simulink model "s3"  (R2025b)
settings: Solver=VariableStepAuto  StartTime=0.0  StopTime=10  RelTol=1e-3
undefined symbols (not defined in the file): X, Y, Z
libraries: nesl_utility x21, sm_lib x20, robotcorelib x1, simulink x1
settings Model: Creator=lucaa  LastModifiedBy=antoniozerbato

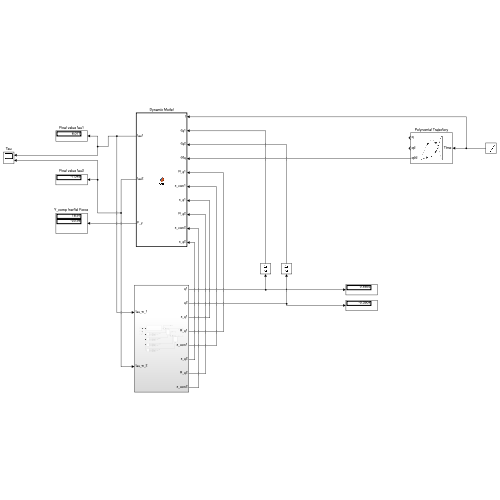
[thumbnail: Simulink's stored preview of the top-level diagram]
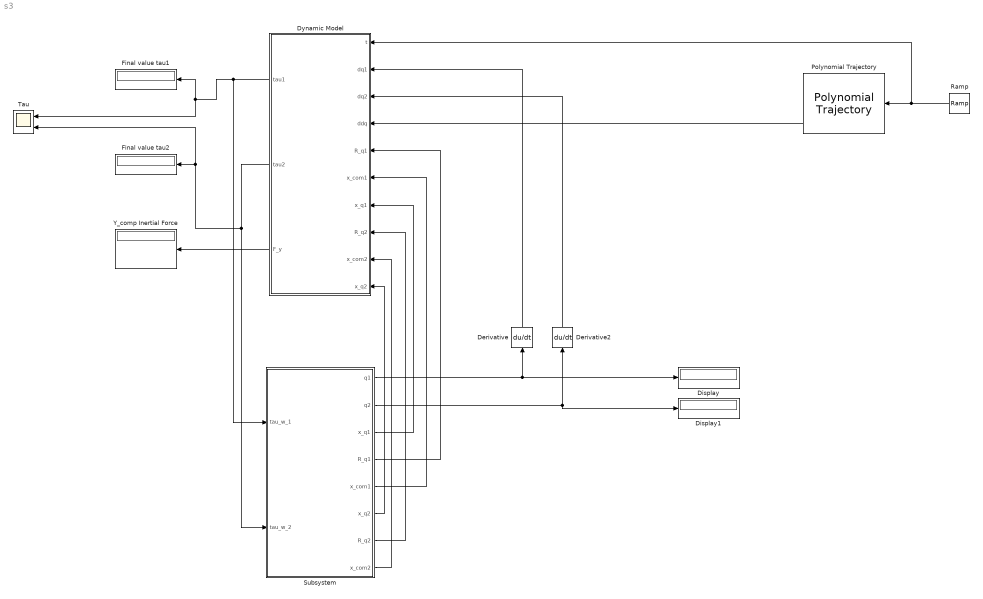
== system s3 ==
  Derivative : Derivative
  Derivative2 : Derivative
  Display : Display
  Display1 : Display
  Dynamic Model : MATLAB Function  TreatAsAtomicUnit=on
  Final value tau1 : Display
  Final value tau2 : Display
  Polynomial Trajectory : robotcorelib/Polynomial Trajectory  WaypointSource=Internal  Waypoints=[pi/36,pi*(4/18);-pi*(3/36),-pi/9]  TimePoints=[0,10]  TimeInterval=[ 1, 4 ]  Method=Cubic Polynomial  ParameterSource=Internal  VelocityBoundaryCondition=zeros( 2,2 )  AccelerationBoundaryCondition=zeros( 2, 5 )  SimulateUsing=Interpreted execution
  Ramp : simulink/Sources/Ramp  slope=1  start=0  InitialOutput=0
  Subsystem : Subsystem
  Tau : Scope  NumInputPorts=2
      settings: ActiveDisplayYMinimum=-0.050415777209954854  ActiveDisplayYMaximum=0.012289469598716157
  "Y_comp Inertial Force " : Display
  wires:
  Dynamic Model/1(tau1) -> Subsystem/1(tau_w_1), Final value tau1/1, Tau/1
  Dynamic Model/2(tau2) -> Subsystem/2(tau_w_2), Final value tau2/1, Tau/2
  Polynomial Trajectory/3 -> Dynamic Model/4(ddq)
  Ramp/1 -> Polynomial Trajectory/1, Dynamic Model/1(t)
  Dynamic Model/3(F_y) -> "Y_comp Inertial Force "/1
  Derivative/1 -> Dynamic Model/2(dq1)
  Derivative2/1 -> Dynamic Model/3(dq2)
  Subsystem/6(x_q2) -> Dynamic Model/10(x_q2)
  Subsystem/8(x_com2) -> Dynamic Model/9(x_com2)
  Subsystem/7(R_q2) -> Dynamic Model/8(R_q2)
  Subsystem/3(x_q1) -> Dynamic Model/7(x_q1)
  Subsystem/1(q1) -> Derivative/1, Display/1
  Subsystem/2(q2) -> Derivative2/1, Display1/1
  Subsystem/5(x_com1) -> Dynamic Model/6(x_com1)
  Subsystem/4(R_q1) -> Dynamic Model/5(R_q1)

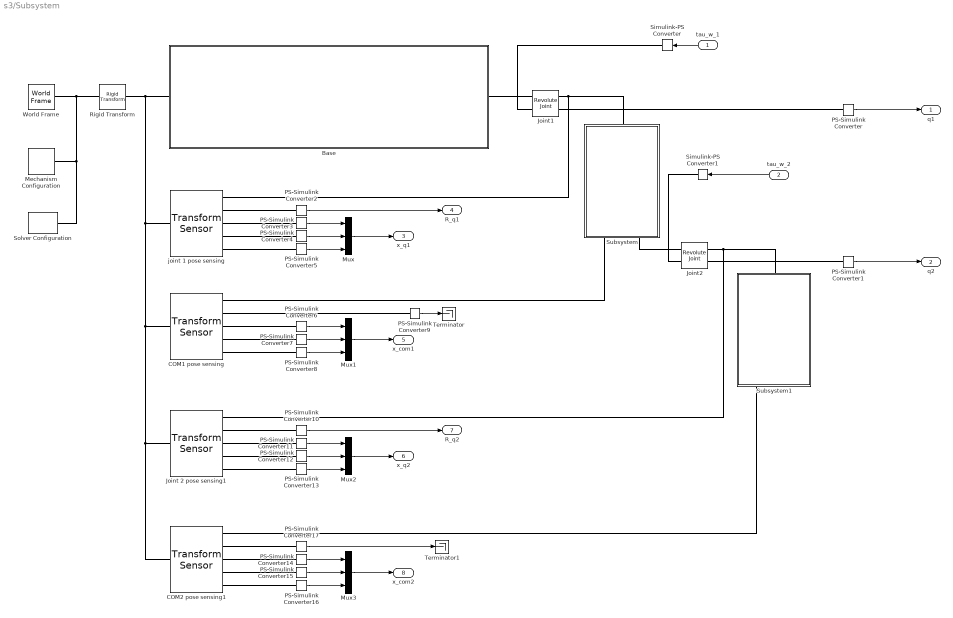
== system s3/Subsystem ==
  tau_w_1 : Inport
  tau_w_2 : Inport  Port=2
  " Joint1" : sm_lib/Joints/Revolute Joint  JointMode=Normal  CompositeWrenchDir=FollowerOnBase  CompositeWrenchFrame=BaseFrame  SenseConstraintForce=off  SenseConstraintTorque=off  SenseTotalForce=off  SenseTotalTorque=off  PositionTargetSpecify=on  PositionTargetPriority=High  PositionTargetValue=5  PositionTargetValueUnits=deg  VelocityTargetSpecify=off  VelocityTargetPriority=High  VelocityTargetValue=0  VelocityTargetValueUnits=deg/s  EquilibriumPosition=0  EquilibriumPositionUnits=deg  SpringStiffness=0  SpringStiffnessUnits=N*m/deg  DampingCoefficient=0  DampingCoefficientUnits=N*m/(deg/s)  LowerLimitSpecify=off  LowerLimitBound=-90  LowerLimitBoundUnits=deg  LowerLimitStiffness=1e4  LowerLimitStiffnessUnits=N*m/deg  LowerLimitDamping=10  LowerLimitDampingUnits=N*m/(deg/s)  LowerLimitTransitionRegionWidth=0.1  LowerLimitTransitionRegionWidthUnits=deg  UpperLimitSpecify=off  UpperLimitBound=90  UpperLimitBoundUnits=deg  UpperLimitStiffness=1e4  UpperLimitStiffnessUnits=N*m/deg  UpperLimitDamping=10  UpperLimitDampingUnits=N*m/(deg/s)  UpperLimitTransitionRegionWidth=0.1  UpperLimitTransitionRegionWidthUnits=deg  TorqueActuationMode=InputTorque  MotionActuationMode=ComputedMotion  SensePosition=on  SenseVelocity=off  SenseAcceleration=off  SenseTorqueForce=off  SenseLowerLimitTorqueForce=off  SenseUpperLimitTorqueForce=off
  " Joint2" : sm_lib/Joints/Revolute Joint  JointMode=Normal  CompositeWrenchDir=FollowerOnBase  CompositeWrenchFrame=BaseFrame  SenseConstraintForce=off  SenseConstraintTorque=off  SenseTotalForce=off  SenseTotalTorque=off  PositionTargetSpecify=on  PositionTargetPriority=High  PositionTargetValue=-15  PositionTargetValueUnits=deg  VelocityTargetSpecify=off  VelocityTargetPriority=High  VelocityTargetValue=0  VelocityTargetValueUnits=deg/s  EquilibriumPosition=0  EquilibriumPositionUnits=deg  SpringStiffness=0  SpringStiffnessUnits=N*m/deg  DampingCoefficient=0  DampingCoefficientUnits=N*m/(deg/s)  LowerLimitSpecify=off  LowerLimitBound=-90  LowerLimitBoundUnits=deg  LowerLimitStiffness=1e4  LowerLimitStiffnessUnits=N*m/deg  LowerLimitDamping=10  LowerLimitDampingUnits=N*m/(deg/s)  LowerLimitTransitionRegionWidth=0.1  LowerLimitTransitionRegionWidthUnits=deg  UpperLimitSpecify=off  UpperLimitBound=90  UpperLimitBoundUnits=deg  UpperLimitStiffness=1e4  UpperLimitStiffnessUnits=N*m/deg  UpperLimitDamping=10  UpperLimitDampingUnits=N*m/(deg/s)  UpperLimitTransitionRegionWidth=0.1  UpperLimitTransitionRegionWidthUnits=deg  TorqueActuationMode=InputTorque  MotionActuationMode=ComputedMotion  SensePosition=on  SenseVelocity=off  SenseAcceleration=off  SenseTorqueForce=off  SenseLowerLimitTorqueForce=off  SenseUpperLimitTorqueForce=off
  Base : Subsystem
  COM1 pose sensing : sm_lib/Frames and Transforms/Transform Sensor  MeasurementFrame=Base  RotationSequence=XYX  SenseAngle=off  SenseAxis=off  SenseQ=off  SenseR=on  SenseRotationSequence=off  SenseOmegaX=off  SenseOmegaY=off  SenseOmegaZ=off  SenseOmega=off  SenseQDot=off  SenseRDot=off  SenseRotationSequenceDot=off  SenseAlphaX=off  SenseAlphaY=off  SenseAlphaZ=off  SenseAlpha=off  SenseQDDot=off  SenseRDDot=off  SenseX=on  SenseY=on  SenseZ=on  SenseXYZ=off  SenseRad=off  SenseAzim=off  SenseDist=off  SenseInc=off  SenseXDot=off  SenseYDot=off  SenseZDot=off  SenseXYZDot=off  SenseRadDot=off  SenseAzimDot=off  SenseDistDot=off  SenseIncDot=off  SenseXDDot=off  SenseYDDot=off  SenseZDDot=off  SenseXYZDDot=off  SenseRadDDot=off  SenseAzimDDot=off  SenseDistDDot=off  SenseIncDDot=off
  COM2 pose sensing1 : sm_lib/Frames and Transforms/Transform Sensor  MeasurementFrame=Base  RotationSequence=XYX  SenseAngle=off  SenseAxis=off  SenseQ=off  SenseR=on  SenseRotationSequence=off  SenseOmegaX=off  SenseOmegaY=off  SenseOmegaZ=off  SenseOmega=off  SenseQDot=off  SenseRDot=off  SenseRotationSequenceDot=off  SenseAlphaX=off  SenseAlphaY=off  SenseAlphaZ=off  SenseAlpha=off  SenseQDDot=off  SenseRDDot=off  SenseX=on  SenseY=on  SenseZ=on  SenseXYZ=off  SenseRad=off  SenseAzim=off  SenseDist=off  SenseInc=off  SenseXDot=off  SenseYDot=off  SenseZDot=off  SenseXYZDot=off  SenseRadDot=off  SenseAzimDot=off  SenseDistDot=off  SenseIncDot=off  SenseXDDot=off  SenseYDDot=off  SenseZDDot=off  SenseXYZDDot=off  SenseRadDDot=off  SenseAzimDDot=off  SenseDistDDot=off  SenseIncDDot=off
  Joint 2 pose sensing1 : sm_lib/Frames and Transforms/Transform Sensor  MeasurementFrame=Base  RotationSequence=XYX  SenseAngle=off  SenseAxis=off  SenseQ=off  SenseR=on  SenseRotationSequence=off  SenseOmegaX=off  SenseOmegaY=off  SenseOmegaZ=off  SenseOmega=off  SenseQDot=off  SenseRDot=off  SenseRotationSequenceDot=off  SenseAlphaX=off  SenseAlphaY=off  SenseAlphaZ=off  SenseAlpha=off  SenseQDDot=off  SenseRDDot=off  SenseX=on  SenseY=on  SenseZ=on  SenseXYZ=off  SenseRad=off  SenseAzim=off  SenseDist=off  SenseInc=off  SenseXDot=off  SenseYDot=off  SenseZDot=off  SenseXYZDot=off  SenseRadDot=off  SenseAzimDot=off  SenseDistDot=off  SenseIncDot=off  SenseXDDot=off  SenseYDDot=off  SenseZDDot=off  SenseXYZDDot=off  SenseRadDDot=off  SenseAzimDDot=off  SenseDistDDot=off  SenseIncDDot=off
  Mechanism Configuration : sm_lib/Utilities/Mechanism Configuration  UniformGravity=Constant  GravityVector=[0 0 -9.80665]  GravityVectorUnits=m/s^2  LinearizationDelta=0.001  JointModeTransitionNonlinearIterations=2
  Mux{,1..3} (4 alike) : Mux  Inputs=3
  PS-Simulink Converter{,1..17} (18 alike) : nesl_utility/PS-Simulink Converter  PhysicalDomain=network_engine_domain  SubClassName=ps_output  LeftPortType=input  RightPortType=output  PseudoPeriodic=off  Frequencies=[]  VectorFormat=inherit  Unit=inherit  AffineConversion=off
  Rigid Transform : sm_lib/Frames and Transforms/Rigid Transform  RotationMethod=AlignedAxes  FollAlignAxisA=+Z  BaseAlignAxisA=-Y  FollAlignAxisB=+X  BaseAlignAxisB=+X  RotationStandardAxis=+Z  RotationAngle=0  RotationAngleUnits=deg  RotationArbitraryAxis=[0 0 1]  RotationSequenceAxes=FollowerAxes  RotationSequence=XYX  RotationSequenceAngles=[0 0 0]  RotationSequenceAnglesUnits=deg  RotationMatrix=[1 0 0;0 1 0;0 0 1]  Quaternion=[1 0 0 0]  TranslationMethod=None  TranslationCartesianOffset=[0 0 0]  TranslationCartesianOffsetUnits=m  TranslationStandardAxis=+Z  TranslationStandardOffset=0  TranslationStandardOffsetUnits=m  TranslationROffset=0  TranslationROffsetUnits=m  TranslationThetaOffset=0  TranslationThetaOffsetUnits=deg  TranslationZOffset=0  TranslationZOffsetUnits=m
  Simulink-PS Converter : nesl_utility/Simulink-PS Converter  PhysicalDomain=network_engine_domain  SubClassName=ps_input  LeftPortType=input  RightPortType=output  PseudoPeriodic=off  Frequencies=[]  NoiseDistribution=none  NoiseParameters=[]  Unit=1  AffineConversion=off  FilteringAndDerivatives=provide  SimscapeFilterOrder=1  InputFilterTimeConstant=0.001  UdotUserProvided=0
  Simulink-PS Converter1 : nesl_utility/Simulink-PS Converter  PhysicalDomain=network_engine_domain  SubClassName=ps_input  LeftPortType=input  RightPortType=output  PseudoPeriodic=off  Frequencies=[]  NoiseDistribution=none  NoiseParameters=[]  Unit=1  AffineConversion=off  FilteringAndDerivatives=provide  SimscapeFilterOrder=1  InputFilterTimeConstant=0.001  UdotUserProvided=0
  Solver Configuration : nesl_utility/Solver Configuration  PhysicalDomain=network_engine_domain  SubClassName=solver  LeftPortType=input  RightPortType=generic  Tones=[]  Harmonics=[]  SimulateNoise=off  Profile=off  UseLocalSampling=off  EnableSwitchedLinearOptims=on  FrequencyDomain=off  UseCCode=off  RelTol=0.001  AbsTol=0.001  MinStep=1e-09  ToWorkspace=off  RevertToSquareIcSolve=off  NumHomotopyIterations=100  PhasorMode=off  PhasorModeNumHarmonics=1  ConsistencySolver=NEWTON_XTOL_AFTER_FTOL  IndexReductionMethod=DerivativeReplacement  DoDC=off  ResidualTolerance=1e-09  ConsistencyTolSource=GLOBAL  ConsistencyAbsTol=0.001  ConsistencyRelTol=0.001  ConsistencyTolFactor=0.001  UseLocalSolver=off  LocalSolverChoice=NE_BACKWARD_EULER_ADVANCER  ResolveIndetEquations=on  FunctionEvalNumThread=1  LocalSolverSampleTime=0.001  DoFixedCost=off  MaxNonlinIter=3  MaxModeIter=2  ComputeImpulses=off  ImpulseIterations=2  LinearAlgebra=auto  LinearAlgebraNumThread=0  EquationFormulation=NE_TIME_EF  DelaysMemoryBudget=1024  AutomaticFiltering=on  FilteringTimeConstant=0.001  PartitionStorageMethod=AS_NEEDED  PartitionMemoryBudget=1024  PartitionMethod=ROBUST  MultibodyUseLocalSolver=off  MultibodyLocalSolverChoice=ODE1  MultibodyLocalSolverSampleTime=0.001
  Subsystem : Subsystem
  Subsystem1 : Subsystem
  Terminator : Terminator
  Terminator1 : Terminator
  World Frame : sm_lib/Frames and Transforms/World Frame
  joint 1 pose sensing : sm_lib/Frames and Transforms/Transform Sensor  MeasurementFrame=Base  RotationSequence=XYX  SenseAngle=off  SenseAxis=off  SenseQ=off  SenseR=on  SenseRotationSequence=off  SenseOmegaX=off  SenseOmegaY=off  SenseOmegaZ=off  SenseOmega=off  SenseQDot=off  SenseRDot=off  SenseRotationSequenceDot=off  SenseAlphaX=off  SenseAlphaY=off  SenseAlphaZ=off  SenseAlpha=off  SenseQDDot=off  SenseRDDot=off  SenseX=on  SenseY=on  SenseZ=on  SenseXYZ=off  SenseRad=off  SenseAzim=off  SenseDist=off  SenseInc=off  SenseXDot=off  SenseYDot=off  SenseZDot=off  SenseXYZDot=off  SenseRadDot=off  SenseAzimDot=off  SenseDistDot=off  SenseIncDot=off  SenseXDDot=off  SenseYDDot=off  SenseZDDot=off  SenseXYZDDot=off  SenseRadDDot=off  SenseAzimDDot=off  SenseDistDDot=off  SenseIncDDot=off
  q1 : Outport
  q2 : Outport  Port=2
  x_q1 : Outport  Port=3
  R_q1 : Outport  Port=4
  x_com1 : Outport  Port=5
  x_q2 : Outport  Port=6
  R_q2 : Outport  Port=7
  x_com2 : Outport  Port=8
  wires:
  PS-Simulink Converter/1 -> q1/1
  PS-Simulink Converter13/1 -> Mux2/3
  PS-Simulink Converter12/1 -> Mux2/2
  PS-Simulink Converter4/1 -> Mux/2
  PS-Simulink Converter9/1 -> Terminator/1
  PS-Simulink Converter11/1 -> Mux2/1
  tau_w_2/1 -> Simulink-PS Converter1/1
  PS-Simulink Converter3/1 -> Mux/1
  PS-Simulink Converter16/1 -> Mux3/3
  Mux3/1 -> x_com2/1
  Mux/1 -> x_q1/1
  PS-Simulink Converter6/1 -> Mux1/1
  PS-Simulink Converter14/1 -> Mux3/1
  PS-Simulink Converter10/1 -> R_q2/1
  Mux1/1 -> x_com1/1
  PS-Simulink Converter5/1 -> Mux/3
  PS-Simulink Converter7/1 -> Mux1/2
  PS-Simulink Converter15/1 -> Mux3/2
  PS-Simulink Converter1/1 -> q2/1
  PS-Simulink Converter2/1 -> R_q1/1
  PS-Simulink Converter17/1 -> Terminator1/1
  tau_w_1/1 -> Simulink-PS Converter/1
  PS-Simulink Converter8/1 -> Mux1/3
  Mux2/1 -> x_q2/1
  connections:
  Rigid Transform/LConn1 -- World Frame/RConn1 -- Mechanism Configuration/RConn1 -- Solver Configuration/RConn1
  Base/LConn1 -- Rigid Transform/RConn1 -- COM2 pose sensing1/LConn1 -- Joint 2 pose sensing1/LConn1 -- COM1 pose sensing/LConn1 -- joint 1 pose sensing/LConn1
  Subsystem/LConn1 -- " Joint1"/RConn1 -- joint 1 pose sensing/RConn1
  Joint 2 pose sensing1/RConn1 -- Subsystem1/LConn1 -- " Joint2"/RConn1
  Joint 2 pose sensing1/RConn4 -- PS-Simulink Converter12/LConn1
  COM1 pose sensing/RConn3 -- PS-Simulink Converter6/LConn1
  " Joint2"/RConn2 -- PS-Simulink Converter1/LConn1
  " Joint2"/LConn2 -- Simulink-PS Converter1/RConn1
  joint 1 pose sensing/RConn2 -- PS-Simulink Converter2/LConn1
  PS-Simulink Converter13/LConn1 -- Joint 2 pose sensing1/RConn5
  COM1 pose sensing/RConn4 -- PS-Simulink Converter7/LConn1
  PS-Simulink Converter5/LConn1 -- joint 1 pose sensing/RConn5
  Subsystem/RConn2 -- " Joint2"/LConn1
  Joint 2 pose sensing1/RConn2 -- PS-Simulink Converter10/LConn1
  COM1 pose sensing/RConn5 -- PS-Simulink Converter8/LConn1
  PS-Simulink Converter17/LConn1 -- COM2 pose sensing1/RConn2
  Joint 2 pose sensing1/RConn3 -- PS-Simulink Converter11/LConn1
  COM2 pose sensing1/RConn5 -- PS-Simulink Converter16/LConn1
  PS-Simulink Converter/LConn1 -- " Joint1"/RConn2
  joint 1 pose sensing/RConn4 -- PS-Simulink Converter4/LConn1
  COM2 pose sensing1/RConn1 -- Subsystem1/RConn1
  COM1 pose sensing/RConn1 -- Subsystem/RConn1
  PS-Simulink Converter9/LConn1 -- COM1 pose sensing/RConn2
  Base/RConn1 -- " Joint1"/LConn1
  " Joint1"/LConn2 -- Simulink-PS Converter/RConn1
  joint 1 pose sensing/RConn3 -- PS-Simulink Converter3/LConn1
  COM2 pose sensing1/RConn3 -- PS-Simulink Converter14/LConn1
  COM2 pose sensing1/RConn4 -- PS-Simulink Converter15/LConn1

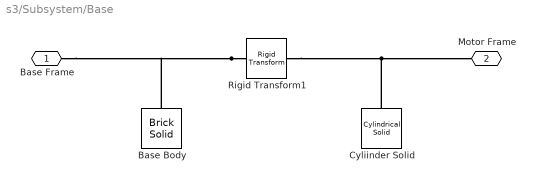
== system s3/Subsystem/Base ==
  " Base Body" : sm_lib/Body Elements/Brick Solid  BrickDimensions=[10 10 1]  BrickDimensionsUnits=cm  ExportEntireGeometry=off  InertiaType=CalculateFromGeometry  BasedOnType=Density  Density=1000  DensityUnits=kg/m^3  Mass=1  MassUnits=kg  CenterOfMass=[0 0 0]  CenterOfMassUnits=m  MomentsOfInertia=[1 1 1]  MomentsOfInertiaUnits=kg*m^2  ProductsOfInertia=[0 0 0]  ProductsOfInertiaUnits=kg*m^2  GraphicType=FromGeometry  MarkerShape=Sphere  MarkerSize=10  GraphicVisPropType=SimpleVisualProperties  GraphicDiffuseColor=[0 0 0]  GraphicOpacity=1  GraphicSpecularColor=[0.5 0.5 0.5 1.0]  GraphicAmbientColor=[0.15 0.15 0.15 1.0]  GraphicEmissiveColor=[0.0 0.0 0.0 1.0]  GraphicShininess=75  DoExposeReferenceFrame=on  SerializedFrames=<Frames/>
  Cyliinder Solid : sm_lib/Body Elements/Cylindrical Solid  CylinderRadius=1.5  CylinderRadiusUnits=cm  CylinderLength=5  CylinderLengthUnits=cm  ExportEntireGeometry=off  InertiaType=CalculateFromGeometry  BasedOnType=Mass  Density=1000  DensityUnits=kg/m^3  Mass=0  MassUnits=kg  CenterOfMass=[0 0 0]  CenterOfMassUnits=m  MomentsOfInertia=[1 1 1]  MomentsOfInertiaUnits=kg*m^2  ProductsOfInertia=[0 0 0]  ProductsOfInertiaUnits=kg*m^2  GraphicType=FromGeometry  MarkerShape=Sphere  MarkerSize=10  GraphicVisPropType=SimpleVisualProperties  GraphicDiffuseColor=[0 0.4941 0.7412]  GraphicOpacity=1  GraphicSpecularColor=[0.5 0.5 0.5 1.0]  GraphicAmbientColor=[0.15 0.15 0.15 1.0]  GraphicEmissiveColor=[0.0 0.0 0.0 1.0]  GraphicShininess=75  DoExposeReferenceFrame=on  SerializedFrames=<Frames/>
  Rigid Transform1 : sm_lib/Frames and Transforms/Rigid Transform  RotationMethod=None  FollAlignAxisA=+Z  BaseAlignAxisA=+X  FollAlignAxisB=+Y  BaseAlignAxisB=+Y  RotationStandardAxis=+Z  RotationAngle=0  RotationAngleUnits=deg  RotationArbitraryAxis=[0 0 1]  RotationSequenceAxes=FollowerAxes  RotationSequence=XYX  RotationSequenceAngles=[0 0 0]  RotationSequenceAnglesUnits=deg  RotationMatrix=[1 0 0;0 1 0;0 0 1]  Quaternion=[1 0 0 0]  TranslationMethod=Cartesian  TranslationCartesianOffset=[0 0 3]  TranslationCartesianOffsetUnits=cm  TranslationStandardAxis=+Z  TranslationStandardOffset=0  TranslationStandardOffsetUnits=m  TranslationROffset=0  TranslationROffsetUnits=m  TranslationThetaOffset=0  TranslationThetaOffsetUnits=deg  TranslationZOffset=0  TranslationZOffsetUnits=m
  Base Frame : PMIOPort  Side=Left
  Motor Frame : PMIOPort  Port=2  Side=Right
  connections:
  Rigid Transform1/LConn1 -- Base Frame/RConn1 -- " Base Body"/RConn1
  Rigid Transform1/RConn1 -- Motor Frame/RConn1 -- Cyliinder Solid/RConn1

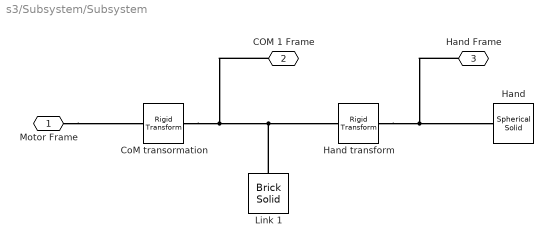
== system s3/Subsystem/Subsystem ==
  " Hand" : sm_lib/Body Elements/Spherical Solid  SphereRadius=1.5  SphereRadiusUnits=cm  ExportEntireGeometry=off  InertiaType=CalculateFromGeometry  BasedOnType=Mass  Density=1000  DensityUnits=kg/m^3  Mass=0  MassUnits=kg  CenterOfMass=[0 0 0]  CenterOfMassUnits=m  MomentsOfInertia=[1 1 1]  MomentsOfInertiaUnits=kg*m^2  ProductsOfInertia=[0 0 0]  ProductsOfInertiaUnits=kg*m^2  GraphicType=FromGeometry  MarkerShape=Sphere  MarkerSize=10  GraphicVisPropType=SimpleVisualProperties  GraphicDiffuseColor=[0.5804 0.1294 0.5725]  GraphicOpacity=1  GraphicSpecularColor=[0.5 0.5 0.5 1.0]  GraphicAmbientColor=[0.15 0.15 0.15 1.0]  GraphicEmissiveColor=[0.0 0.0 0.0 1.0]  GraphicShininess=75  DoExposeReferenceFrame=on  SerializedFrames=<Frames/>
  CoM transormation : sm_lib/Frames and Transforms/Rigid Transform  RotationMethod=None  FollAlignAxisA=+X  BaseAlignAxisA=+Y  FollAlignAxisB=+Y  BaseAlignAxisB=+Z  RotationStandardAxis=+Z  RotationAngle=0  RotationAngleUnits=deg  RotationArbitraryAxis=[0 0 1]  RotationSequenceAxes=FollowerAxes  RotationSequence=XYX  RotationSequenceAngles=[0 0 0]  RotationSequenceAnglesUnits=deg  RotationMatrix=[1 0 0;0 1 0;0 0 1]  Quaternion=[1 0 0 0]  TranslationMethod=Cartesian  TranslationCartesianOffset=[10 0 0]  TranslationCartesianOffsetUnits=cm  TranslationStandardAxis=+Z  TranslationStandardOffset=0  TranslationStandardOffsetUnits=m  TranslationROffset=0  TranslationROffsetUnits=m  TranslationThetaOffset=0  TranslationThetaOffsetUnits=deg  TranslationZOffset=0  TranslationZOffsetUnits=m
  Hand transform : sm_lib/Frames and Transforms/Rigid Transform  RotationMethod=AlignedAxes  FollAlignAxisA=+X  BaseAlignAxisA=+Z  FollAlignAxisB=-Y  BaseAlignAxisB=+Y  RotationStandardAxis=+Z  RotationAngle=0  RotationAngleUnits=deg  RotationArbitraryAxis=[0 0 1]  RotationSequenceAxes=FollowerAxes  RotationSequence=XYX  RotationSequenceAngles=[0 0 0]  RotationSequenceAnglesUnits=deg  RotationMatrix=[1 0 0;0 1 0;0 0 1]  Quaternion=[1 0 0 0]  TranslationMethod=Cartesian  TranslationCartesianOffset=[10 0 0]  TranslationCartesianOffsetUnits=cm  TranslationStandardAxis=+Z  TranslationStandardOffset=0  TranslationStandardOffsetUnits=m  TranslationROffset=0  TranslationROffsetUnits=m  TranslationThetaOffset=0  TranslationThetaOffsetUnits=deg  TranslationZOffset=0  TranslationZOffsetUnits=m
  Link 1 : sm_lib/Body Elements/Brick Solid  BrickDimensions=[20 1 1]  BrickDimensionsUnits=cm  ExportEntireGeometry=off  InertiaType=CalculateFromGeometry  BasedOnType=Mass  Density=1000  DensityUnits=kg/m^3  Mass=2.5  MassUnits=kg  CenterOfMass=[0 0 0]  CenterOfMassUnits=m  MomentsOfInertia=[1 1 1]  MomentsOfInertiaUnits=kg*m^2  ProductsOfInertia=[0 0 0]  ProductsOfInertiaUnits=kg*m^2  GraphicType=FromGeometry  MarkerShape=Sphere  MarkerSize=10  GraphicVisPropType=SimpleVisualProperties  GraphicDiffuseColor=[0.5647 0.5647 0.5647]  GraphicOpacity=1  GraphicSpecularColor=[0.5 0.5 0.5 1.0]  GraphicAmbientColor=[0.15 0.15 0.15 1.0]  GraphicEmissiveColor=[0.0 0.0 0.0 1.0]  GraphicShininess=75  DoExposeReferenceFrame=on  SerializedFrames=<Frames/>
  Motor Frame : PMIOPort  Side=Left
  " COM 1 Frame" : PMIOPort  Port=2  Side=Right
  Hand Frame : PMIOPort  Port=3  Side=Right
  connections:
  CoM transormation/RConn1 -- " COM 1 Frame"/RConn1 -- Link 1/RConn1 -- Hand transform/LConn1
  Hand transform/RConn1 -- Hand Frame/RConn1 -- " Hand"/RConn1
  Motor Frame/RConn1 -- CoM transormation/LConn1

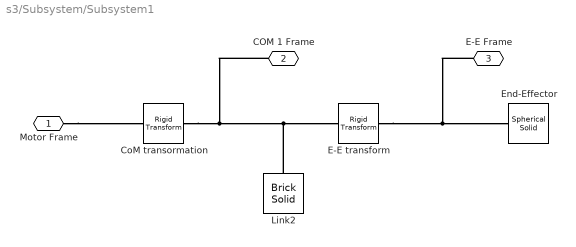
== system s3/Subsystem/Subsystem1 ==
  " End-Effector" : sm_lib/Body Elements/Spherical Solid  SphereRadius=1.5  SphereRadiusUnits=cm  ExportEntireGeometry=off  InertiaType=CalculateFromGeometry  BasedOnType=Mass  Density=1000  DensityUnits=kg/m^3  Mass=0  MassUnits=kg  CenterOfMass=[0 0 0]  CenterOfMassUnits=m  MomentsOfInertia=[1 1 1]  MomentsOfInertiaUnits=kg*m^2  ProductsOfInertia=[0 0 0]  ProductsOfInertiaUnits=kg*m^2  GraphicType=FromGeometry  MarkerShape=Sphere  MarkerSize=10  GraphicVisPropType=SimpleVisualProperties  GraphicDiffuseColor=[0.5804 0.1294 0.5725]  GraphicOpacity=1  GraphicSpecularColor=[0.5 0.5 0.5 1.0]  GraphicAmbientColor=[0.15 0.15 0.15 1.0]  GraphicEmissiveColor=[0.0 0.0 0.0 1.0]  GraphicShininess=75  DoExposeReferenceFrame=on  SerializedFrames=<Frames/>
  CoM transormation : sm_lib/Frames and Transforms/Rigid Transform  RotationMethod=None  FollAlignAxisA=+X  BaseAlignAxisA=+Y  FollAlignAxisB=+Y  BaseAlignAxisB=+Z  RotationStandardAxis=+Z  RotationAngle=0  RotationAngleUnits=deg  RotationArbitraryAxis=[0 0 1]  RotationSequenceAxes=FollowerAxes  RotationSequence=XYX  RotationSequenceAngles=[0 0 0]  RotationSequenceAnglesUnits=deg  RotationMatrix=[1 0 0;0 1 0;0 0 1]  Quaternion=[1 0 0 0]  TranslationMethod=Cartesian  TranslationCartesianOffset=[10/2 0 0]  TranslationCartesianOffsetUnits=cm  TranslationStandardAxis=+Z  TranslationStandardOffset=0  TranslationStandardOffsetUnits=m  TranslationROffset=0  TranslationROffsetUnits=m  TranslationThetaOffset=0  TranslationThetaOffsetUnits=deg  TranslationZOffset=0  TranslationZOffsetUnits=m
  E-E transform : sm_lib/Frames and Transforms/Rigid Transform  RotationMethod=None  FollAlignAxisA=+X  BaseAlignAxisA=+Y  FollAlignAxisB=+Y  BaseAlignAxisB=+Z  RotationStandardAxis=+Z  RotationAngle=0  RotationAngleUnits=deg  RotationArbitraryAxis=[0 0 1]  RotationSequenceAxes=FollowerAxes  RotationSequence=XYX  RotationSequenceAngles=[0 0 0]  RotationSequenceAnglesUnits=deg  RotationMatrix=[1 0 0;0 1 0;0 0 1]  Quaternion=[1 0 0 0]  TranslationMethod=Cartesian  TranslationCartesianOffset=[10/2 0 0]  TranslationCartesianOffsetUnits=cm  TranslationStandardAxis=+Z  TranslationStandardOffset=0  TranslationStandardOffsetUnits=m  TranslationROffset=0  TranslationROffsetUnits=m  TranslationThetaOffset=0  TranslationThetaOffsetUnits=deg  TranslationZOffset=0  TranslationZOffsetUnits=m
  Link2 : sm_lib/Body Elements/Brick Solid  BrickDimensions=[10 1 1]  BrickDimensionsUnits=cm  ExportEntireGeometry=off  InertiaType=CalculateFromGeometry  BasedOnType=Mass  Density=1000  DensityUnits=kg/m^3  Mass=3  MassUnits=kg  CenterOfMass=[0 0 0]  CenterOfMassUnits=m  MomentsOfInertia=[1 1 1]  MomentsOfInertiaUnits=kg*m^2  ProductsOfInertia=[0 0 0]  ProductsOfInertiaUnits=kg*m^2  GraphicType=FromGeometry  MarkerShape=Sphere  MarkerSize=10  GraphicVisPropType=SimpleVisualProperties  GraphicDiffuseColor=[0.5647 0.5647 0.5647]  GraphicOpacity=1  GraphicSpecularColor=[0.5 0.5 0.5 1.0]  GraphicAmbientColor=[0.15 0.15 0.15 1.0]  GraphicEmissiveColor=[0.0 0.0 0.0 1.0]  GraphicShininess=75  DoExposeReferenceFrame=on  SerializedFrames=<Frames/>
  Motor Frame : PMIOPort  Side=Left
  " COM 1 Frame" : PMIOPort  Port=2  Side=Right
  E-E Frame : PMIOPort  Port=3  Side=Right
  connections:
  CoM transormation/RConn1 -- " COM 1 Frame"/RConn1 -- Link2/RConn1 -- E-E transform/LConn1
  E-E transform/RConn1 -- E-E Frame/RConn1 -- " End-Effector"/RConn1
  Motor Frame/RConn1 -- CoM transormation/LConn1

== matlab function s3/Dynamic Model ==
  data: t input; tau1 output; tau2 output; dq1 input; dq2 input; ddq input; R_q1 input; x_com1 input; x_q1 input; R_q2 input; x_com2 input; x_q2 input; F_y output
%IMPLEMENTATION OF INVVERSE DYNAMIC PORBLEM
function [tau1, tau2, F_y]   = fcn(t, dq1, dq2, ddq, R_q1, x_com1, x_q1, R_q2, x_com2, x_q2)


%% DATA INITALIZATION

dq=[dq1;dq2];

m1 = 2.5;
m2 = 3;
m = [m1; m2];    % mass vector

w_0 = [0;0;0];      
dw_0 = [0;0;0];

g = [0;9.80665;0];
n = 2;               %number link

l1 = 0.2;
l2 = 0.1;
l = [l1; l2];    %link lenght vector

bc_I = zeros(3,3,n); %inertial operator

k = zeros(3,n);      %z-axis

R = zeros(3,3,n+1);      % rotation matrices from i-1 to i
R(:,:,1) = R_q1';        % from 0 to 1
R(:,:,2) = R_q2'*R_q1;   % rotation from 1 to 2 
R(:,:,n+1) = eye(3);     % end effector

for i=1:n
    %inertial operator
    bc_I(:,:,i) = zeros(3);
    %bc_I(2,2, i) = (1/12) * m(i) * l(i)^2;
    bc_I(3,3, i) = (1/12) * m(i) * l(i)^2;

    k(:,i) = [0;0;1];    %z-axis
end

% centers of mass i vectors wrt base i
b_x_com = zeros(3, n);
b_x_com(:,1) = R_q1' *(x_com1 - x_q1);
b_x_com(:,2) = R_q2' *(x_com2 - x_q2);

% r_i_prev_i: vettore che va dal giunto i-1 al giunto i, espresso nel frame i-1
x_rel = zeros(3, n+1);

x_rel(:,1) = [0;0;0.05];     % from base to joint 1
x_rel(:,2) = [0.2;0;0];     % from joint 1 to joint2
x_rel(:,3) = [0.0;0;0];     % from joint 2 to joint 3

% data for backward and forward computation
w_i_0 = zeros(3,n);
wdot_i_0 = zeros(3,n);
vdot_i_0 = zeros(3,n);
vdot_Ci_0 = zeros(3,n);
F_i = zeros(3,n);
N_i = zeros(3,n);
f = zeros(3, n+1);          %forces of joint i acting on i-1
ni = zeros(3, n+1);         %momentun of joint i acting on i-1

tau = zeros(1,n);

%% FORWARD PROPAGATION

for i=1:n

    if i==1
        w_prev = w_0;
        wdot_prev = dw_0;
        vdot_prev = g; 
    else
        w_prev = w_i_0(:, i-1);
        wdot_prev = wdot_i_0(:, i-1);
        vdot_prev = vdot_i_0(:, i-1);
    end

    w_i_0(:,i) = R(:,:,i)* w_prev + dq(i)*k(:,i);
    % Angolar Acceleration
    wdot_i_0(:,i) = R(:,:,i) * wdot_prev+cross(R(:,:,i)*w_prev, dq(i)*k(:,i))+ ddq(i)* k(:,i);
    % Linear Acceleration
    vdot_i_0(:,i) = R(:,:,i) *(cross(wdot_prev, x_rel(:,i)) + cross(w_prev, cross(w_prev,x_rel(:,i))) + vdot_prev );
    % Linear Acceleration of COM
    vdot_Ci_0(:,i) = cross(wdot_i_0(:,i), b_x_com(:,i)) + cross(w_i_0(:,i), cross(w_i_0(:,i),b_x_com(:,i))) +vdot_i_0(:,i);
    % Force on COM, newton law (intertial force)
    F_i(:,i) = m(i)*vdot_Ci_0(:,i);
    % Torque on COM, newton-euler law (intertial mementum)
    N_i(:,i) = bc_I(:,:,i) * wdot_i_0(:,i) + cross(w_i_0(:,i),bc_I(:,:,i)*w_i_0(:,i));

end

%% BACKWARD PROPAGATION
for i=n:-1:1
    % Force acting on joint i (intertial + force acting on joint i+1)
    f(:,i) = R(:,:,i+1)'*f(:,i+1) + F_i(:,i);
    % Torque action on joint i (inertial + momentum acting on joint i+1 + angular momentum of the inertial     
    ni(:,i) = N_i(:,i) + R(:,:,i+1)'* ni(:,i+1) + cross(b_x_com(:,i), F_i(:,i) ) + cross(x_rel(:,i+1), R(:,:,i+1)'*f(:,i+1)); %ricordarsi di portare tutto rispetto a i
 
    tau(i) = ni(:,i)'*k(:,i);

end

F_y = [0,0];
F_y(1) = F_i(2,1);
F_y(2) = F_i(2,2);


tau1 = tau(1);
tau2 = tau(2);
